simulink model "ApproxPDcontroller"  (R2018a)
settings: Solver=FixedStepAuto  StartTime=0.0  StopTime=10.0  FixedStep=0.001  RelTol=1e-3
libraries: cstblocks x2
settings Model: Creator=ayush2  LastModifiedBy=ayush2

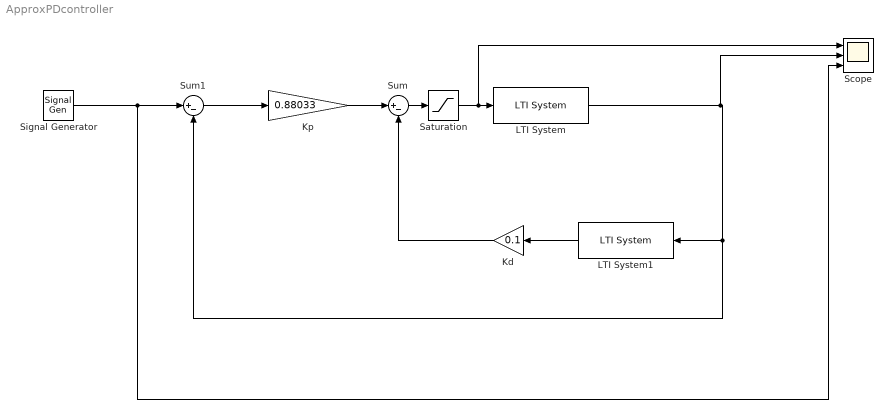
== system ApproxPDcontroller ==
  Kd : Gain  Gain=0.1
  Kp : Gain  Gain=0.88033
  LTI System : cstblocks/LTI System  sys=mydtf  IC=[]
  LTI System1 : cstblocks/LTI System  sys=mydstf  IC=[]
  Saturation : Saturate  UpperLimit=10  LowerLimit=-10
  Scope : Scope  NumInputPorts=3
  Signal Generator : SignalGenerator  WaveForm=square  Frequency=0.25
  Sum : Sum  Inputs=|+-
  Sum1 : Sum  Inputs=|+-
  wires:
  Sum/1 -> Saturation/1
  Kp/1 -> Sum/1
  LTI System/1 -> Scope/2, LTI System1/1, Sum1/2
  LTI System1/1 -> Kd/1
  Kd/1 -> Sum/2
  Sum1/1 -> Kp/1
  Signal Generator/1 -> Scope/3, Sum1/1
  Saturation/1 -> Scope/1, LTI System/1
